simulink model "openloop_model"  (R2024a)
settings: Solver=ode45  StartTime=0.0  StopTime=20.0  FixedStep=0.001  MaxStep=0.001  RelTol=1e-3
undefined symbols (not defined in the file): Kp, Td, Ti
libraries: cstblocks x2
settings Model: Creator=thoma  LastModifiedBy=Flo

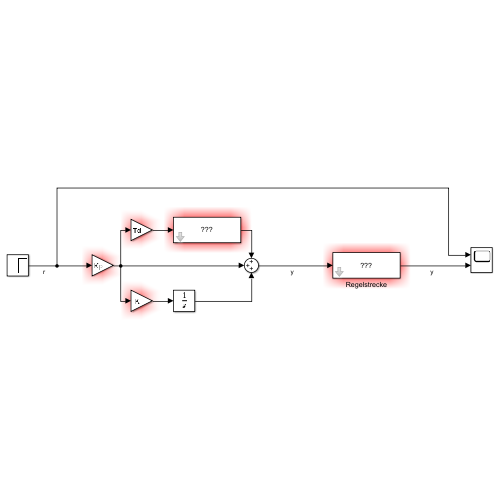
[thumbnail: Simulink's stored preview of the top-level diagram]
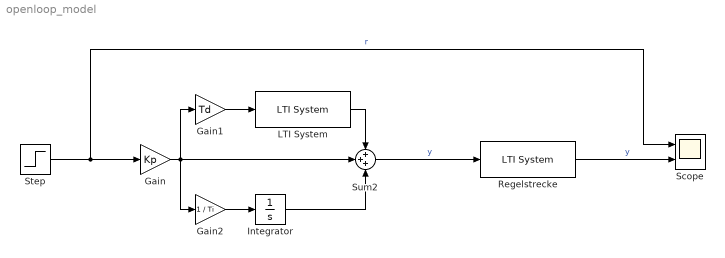
== system openloop_model ==
  Gain : Gain  Gain=Kp
  Gain1 : Gain  Gain=Td
  Gain2 : Gain  Gain=1 / Ti
  Integrator : Integrator
  LTI System : cstblocks/LTI System  sys=F  IC=[]  PadeOrder=0
  Regelstrecke : cstblocks/LTI System  sys=G  IC=[]  PadeOrder=0
  Scope : Scope  NumInputPorts=2
  Step : Step  Time=0  SampleTime=0
  Sum2 : Sum  Inputs=+++
  wires:
  Step/1 -> Gain/1, Scope/1  "r"
  Regelstrecke/1 -> Scope/2  "y"
  Sum2/1 -> Regelstrecke/1  "y"
  Gain/1 -> Sum2/2, Gain1/1, Gain2/1
  Gain1/1 -> LTI System/1
  Gain2/1 -> Integrator/1
  Integrator/1 -> Sum2/3
  LTI System/1 -> Sum2/1
